simulink model "test_loi_commande"  (R2013a)
settings: Solver=FixedStepDiscrete  StartTime=0.0  StopTime=15  FixedStep=0.01  RelTol=1e-3
libraries: ardrone_lib x2
settings Model: Creator=Arnaud  LastModifiedBy=Arnaud
settings OptimizationCC: InitFltsAndDblsToZero=on  OptimizeModelRefInitCode=on  LifeSpan=1
settings RTWCC: SystemTargetFile=ardrone.tlc  TemplateMakefile=ardrone.tmf  Description=AR.Drone_v2  ProcessScript=ardrone_make_rtw_hook  TargetLang=C++
settings CodeAppCC: IgnoreCustomStorageClasses=off
settings STFCustomTargetCC: GenerateSampleERTMain=on  ModelReferenceCompliant=off  CombineOutputUpdateFcns=on  ERTCustomFileBanners=on  SupportContinuousTime=off  SupportNonInlinedSFcns=off  MATLABClassNameForMDSCustomization=Simulink.SoftwareTarget.ERTCustomization  SystemTargetFile=ardrone.tlc
settings ERTTargetCC: ModelReferenceCompliant=off  ParMdlRefBuildCompliant=off  CompOptLevelCompliant=off  ConcurrentExecutionCompliant=off  ERTFirstTimeCompliant=off  ModelStepFunctionPrototypeControlCompliant=off  CPPClassGenCompliant=off  InlinedParameterPlacement=Hierarchical  ERTSrcFileBannerTemplate=example_banner.tlc  ERTHdrFileBannerTemplate=example_banner.tlc  ERTCustomFileTemplate=ardrone_file_process.tlc

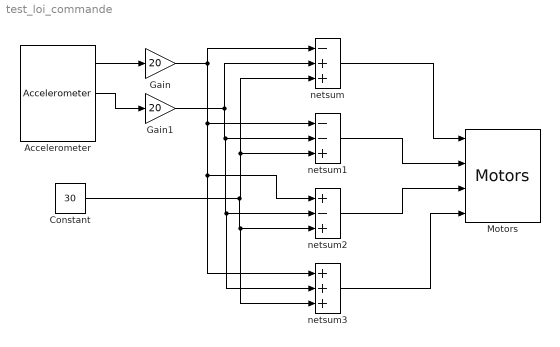
== system test_loi_commande ==
  Accelerometer : ardrone_lib/Accelerometer  SystemSampleTime=-1
  Constant : Constant  Value=30  OutDataTypeStr=single
  Gain : Gain  Gain=20
  Gain1 : Gain  Gain=20
  Motors : ardrone_lib/Motors  SystemSampleTime=-1
  netsum : Sum  Inputs=-++  SaturateOnIntegerOverflow=on  InputSameDT=on  OutDataTypeStr=Inherit: Same as first input
  netsum1 : Sum  Inputs=--+  SaturateOnIntegerOverflow=on  InputSameDT=on  OutDataTypeStr=Inherit: Same as first input
  netsum2 : Sum  Inputs=+-+  SaturateOnIntegerOverflow=on  InputSameDT=on  OutDataTypeStr=Inherit: Same as first input
  netsum3 : Sum  Inputs=+++  SaturateOnIntegerOverflow=on  InputSameDT=on  OutDataTypeStr=Inherit: Same as first input
  wires:
  Accelerometer/1 -> Gain/1
  Gain/1 -> netsum3/1, netsum2/1, netsum1/1, netsum/1
  Constant/1 -> netsum3/3, netsum2/3, netsum1/3, netsum/3
  Accelerometer/2 -> Gain1/1
  Gain1/1 -> netsum3/2, netsum2/2, netsum1/2, netsum/2
  netsum1/1 -> Motors/2
  netsum2/1 -> Motors/3
  netsum3/1 -> Motors/4
  netsum/1 -> Motors/1
